simulink model "s0613"  (Simulink 6.0)
settings: Solver=ode45  SolverMode=SingleTasking  StartTime=0.0  StopTime=10  MaxStep=.1  RelTol=1e-3  AbsTol=1e-6
values from neighbouring files (symbols this model uses):
  b0 = omega0*((2*rP/l)*cos(phi0)+sin(2*phi0))    [m0218a.m]    (also in m0218e.m; m0251.m = 10; m0252.m = -10)
  Kpr = 10    [m0108d.m]    (also in m0109b.m = 1; m0113c.m; m0404Bsp.m = 3)
  T = 1    [m0304.m]
undefined symbols (not defined in the file or in its folder): b1, b2, Tn
settings Model: LastModifiedBy=Froriep
settings DataIOCC: LimitDataPoints=off  SaveOutput=off  TimeSaveName=t
settings OptimizationCC: BooleanDataType=off
settings DebuggingCC: SolverPrmCheckMsg=none
settings HardwareCC: TargetUnknown=on
settings STFCustomTargetCC: TargetFcnLib=ansi_tfl_tmw.mat  GenFloatMathFcnCalls=ANSI_C  ModelReferenceCompliant=off  SystemTargetFile=grt.tlc

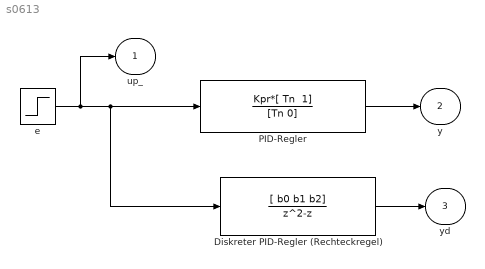
== system s0613 ==
  Diskreter PID-Regler (Rechteckregel) : DiscreteTransferFcn  Numerator=[ b0 b1 b2]  Denominator=[1 -1 0]  SampleTime=T
  PID-Regler : TransferFcn  Numerator="Kpr*[ Tn  1]"  Denominator=[Tn 0]
  e : Step  Time=0.0  SampleTime=0
  up_ : Outport
  y : Outport  Port=2
  yd : Outport  Port=3
  wires:
  e/1 -> up_/1, PID-Regler/1, Diskreter PID-Regler (Rechteckregel)/1
  PID-Regler/1 -> y/1
  Diskreter PID-Regler (Rechteckregel)/1 -> yd/1
